simulink model "regulator"  (Simulink 7.5)
settings: Solver=ode45  StartTime=0.0  StopTime=40.0  RelTol=1e-3
libraries: simulink_need_slupdate x1
settings Model: Creator=Bartek  LastModifiedBy=dotevo
settings DebuggingCC: StrictBusMsg=Warning

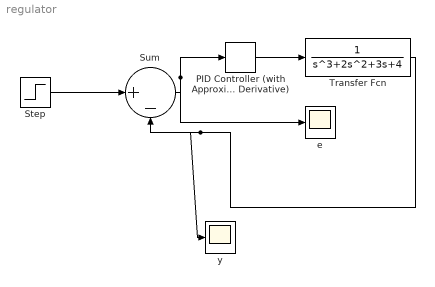
== system regulator ==
  PID Controller (with Approximate Derivative) : simulink_need_slupdate/PID Controller (with Approximate Derivative)  SystemSampleTime=-1  P=9.35  I=1  D=4  N=100
  Step : Step  SampleTime=0
  Sum : Sum  Inputs=|+-  OutDataType=fixdt(1, 16)  OutScaling=2^0
  Transfer Fcn : TransferFcn  Denominator=[1 2 3 4]
  e : Scope
  y : Scope
  wires:
  Step/1 -> Sum/1
  Sum/1 -> PID Controller (with Approximate Derivative)/1, e/1
  PID Controller (with Approximate Derivative)/1 -> Transfer Fcn/1
  Transfer Fcn/1 -> Sum/2, y/1
